simulink model "EPWM_test2_21b"  (R2021b)
settings: Solver=VariableStepAuto  StartTime=0.0  StopTime=10.0  RelTol=1e-3
libraries: simulink x1
settings Model: Creator=Maxwill  LastModifiedBy=Maxwill
settings DebuggingCC: UnconnectedInputMsg=none  UnconnectedOutputMsg=none  UnconnectedLineMsg=none
settings RTWCC: DLArmComputeVersion=20.02.1

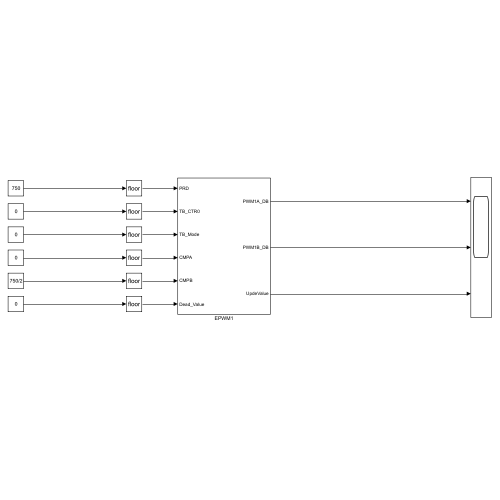
[thumbnail: Simulink's stored preview of the top-level diagram]
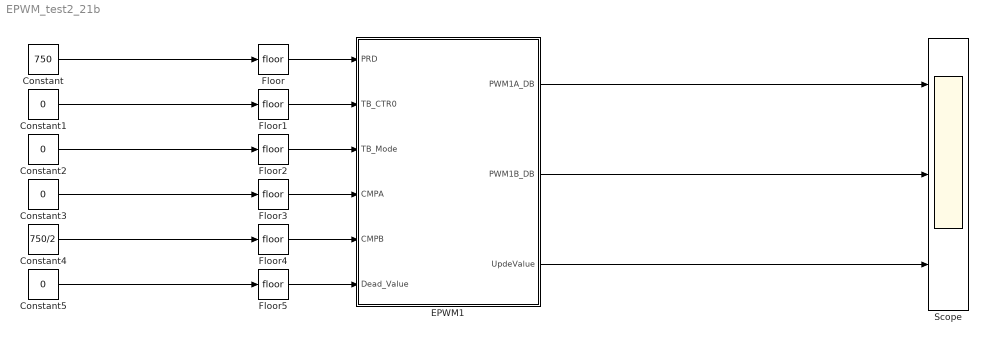
== system EPWM_test2_21b ==
  Constant : Constant  Value=750
  Constant{1..3,5} (4 alike) : Constant  Value=0
  Constant4 : Constant  Value=750/2
  EPWM1 : Subsystem
  Floor{,1..5} (6 alike) : Rounding
  Scope : Scope  NumInputPorts=3
  wires:
  Floor5/1 -> EPWM1/6(Dead_Value)
  EPWM1/1(PWM1A_DB) -> Scope/1
  Constant2/1 -> Floor2/1
  Floor/1 -> EPWM1/1(PRD)
  Constant3/1 -> Floor3/1
  Constant1/1 -> Floor1/1
  Floor3/1 -> EPWM1/4(CMPA)
  EPWM1/3(UpdeValue) -> Scope/3
  Constant/1 -> Floor/1
  Constant4/1 -> Floor4/1
  Constant5/1 -> Floor5/1
  Floor2/1 -> EPWM1/3(TB_Mode)
  Floor1/1 -> EPWM1/2(TB_CTR0)
  EPWM1/2(PWM1B_DB) -> Scope/2
  Floor4/1 -> EPWM1/5(CMPB)

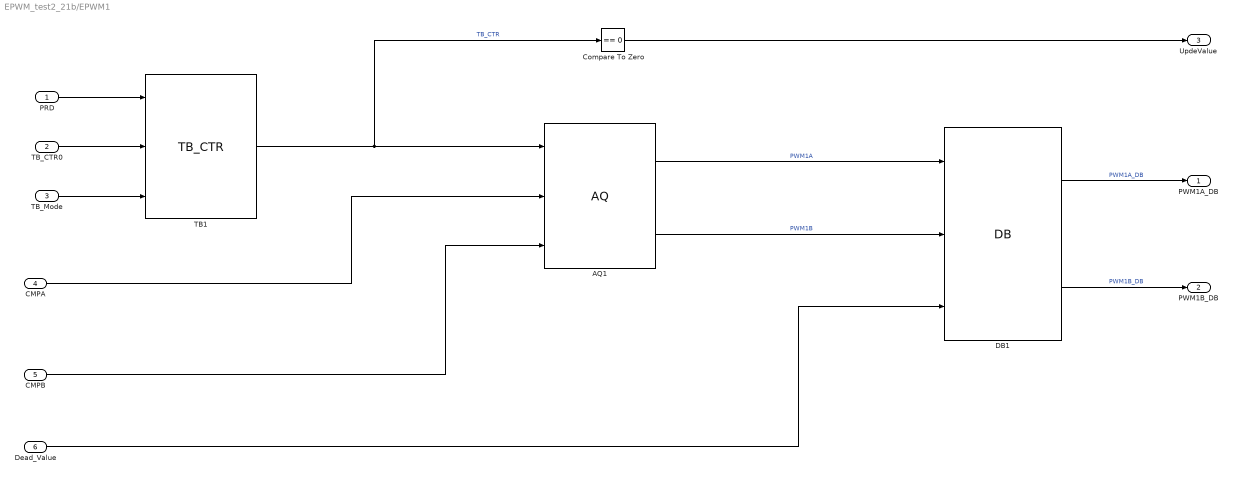
== system EPWM_test2_21b/EPWM1 ==
  PRD : Inport
  TB_CTR0 : Inport  Port=2
  TB_Mode : Inport  Port=3
  CMPA : Inport  Port=4
  CMPB : Inport  Port=5
  Dead_Value : Inport  Port=6
  AQ1 : S-Function  FunctionName=AQ  Parameters=1/(150e6)  SFunctionDeploymentMode=off  EnableBusSupport=off
      mask Display:
      | port_label('input',1,'TB_CTR');
      | port_label('input',2,'CMPA');
      | port_label('input',3,'CMPB');
      | port_label('output',1,'PWMA');
      | port_label('output',2,'PWMB');
  Compare To Zero : simulink/Logic and Bit Operations/Compare To Zero  relop===  OutDataTypeStr=boolean
  DB1 : S-Function  FunctionName=DB  Parameters=1/(150e6)  SFunctionDeploymentMode=off  EnableBusSupport=off
      mask Display:
      | port_label('input',1,'PWMA');
      | port_label('input',2,'PWMB');
      | port_label('input',3,'Dead_Value');
      | port_label('output',1,'PWMA_DB');
      | port_label('output',2,'PWMB_DB');
  TB1 : S-Function  FunctionName=TB_CTR  Parameters=1/(150e6)  SFunctionDeploymentMode=off  EnableBusSupport=off
      mask Display:
      | port_label('input',1,'PRD');
      | port_label('input',2,'TB_CTR_O');
      | port_label('input',3,'TB_Mode');
      | port_label('output',1,'TB_CTR');
  PWM1A_DB : Outport
  PWM1B_DB : Outport  Port=2
  UpdeValue : Outport  Port=3
  wires:
  CMPA/1 -> AQ1/2
  TB1/1 -> Compare To Zero/1, AQ1/1  "TB_CTR"
  CMPB/1 -> AQ1/3
  TB_CTR0/1 -> TB1/2
  TB_Mode/1 -> TB1/3
  AQ1/2 -> DB1/2  "PWM1B"
  PRD/1 -> TB1/1
  DB1/1 -> PWM1A_DB/1  "PWM1A_DB"
  AQ1/1 -> DB1/1  "PWM1A"
  DB1/2 -> PWM1B_DB/1  "PWM1B_DB"
  Dead_Value/1 -> DB1/3
  Compare To Zero/1 -> UpdeValue/1
